simulink model "gm_ZynqBF_2tx_fpga"  (R2018b)
settings: Solver=FixedStepDiscrete  StartTime=0.0  StopTime=10.0  FixedStep=(1/420e3)/128  RelTol=1e-3
undefined symbols (not defined in the file or in its folder): a, b, c
libraries: hdlsllib x873, simulink x349
(part 3 of 40)

== system gm_ZynqBF_2tx_fpga/channel_estimator/gs_selector ==
  pd1 : Inport  OutDataTypeStr=boolean  PortDimensions=1  SampleTime=1.86011904761905e-08
  pd2 : Inport  Port=2  OutDataTypeStr=boolean  PortDimensions=1  SampleTime=1.86011904761905e-08
  en : Inport  Port=3  OutDataTypeStr=boolean  PortDimensions=1  SampleTime=1.86011904761905e-08
  Delay{1..5} (5 alike) : Delay  DelayLength=double(1)  InitialCondition=0  InputProcessing=Inherited  SampleTime=1.86011904761905e-08
  Switch1 : Switch  Criteria=u2 ~= 0  Threshold=double(0)  OutDataTypeStr=boolean  SampleTime=1.86011904761905e-08
  concatenate : Concatenate
  gs_sel : Outport
  wires:
  pd1/1 -> Delay1/1
  pd2/1 -> Delay2/1
  en/1 -> Delay4/1
  Delay1/1 -> concatenate/1
  Delay2/1 -> concatenate/2
  Delay3/1 -> gs_sel/1
  Delay4/1 -> Switch1/2
  Delay5/1 -> Switch1/3
  Switch1/1 -> Delay5/1, Delay3/1
  concatenate/1 -> Switch1/1

== system gm_ZynqBF_2tx_fpga/channel_estimator/in_fifo ==
  rxi_in : Inport  OutDataTypeStr=fixdt(1, 16, 15)  PortDimensions=1  SampleTime=2.38095238095238e-06
  rxq_in : Inport  Port=2  OutDataTypeStr=fixdt(1, 16, 15)  PortDimensions=1  SampleTime=2.38095238095238e-06
  rxv_in : Inport  Port=3  OutDataTypeStr=boolean  PortDimensions=1  SampleTime=2.38095238095238e-06
  pd_en : Inport  Port=4  OutDataTypeStr=boolean  PortDimensions=1  SampleTime=1.86011904761905e-08
  cf_en : Inport  Port=5  OutDataTypeStr=boolean  PortDimensions=1  SampleTime=1.86011904761905e-08
  Delay : Delay  DelayLength=double(1)  InitialCondition=0  InputProcessing=Inherited  SampleTime=2.38095238095238e-06
  Delay1 : Delay  DelayLength=double(1)  InitialCondition=0  InputProcessing=Inherited  SampleTime=2.38095238095238e-06
  Delay4 : Delay  DelayLength=double(2)  InitialCondition=0  InputProcessing=Inherited  SampleTime=1.86011904761905e-08
  Delay5 : Delay  DelayLength=double(1)  InitialCondition=0  InputProcessing=Inherited  SampleTime=1.86011904761905e-08
  Logical Operator : Logic  AllPortsSameDT=off  OutDataTypeStr=boolean  SampleTime=1.86011904761905e-08
  Logical Operator1 : Logic  AllPortsSameDT=off  OutDataTypeStr=boolean  SampleTime=2.38095238095238e-06
  Logical Operator2 : Logic  AllPortsSameDT=off  OutDataTypeStr=boolean  SampleTime=1.86011904761905e-08
  Logical Operator3 : Logic  Operator=NOR  AllPortsSameDT=off  OutDataTypeStr=boolean  SampleTime=1.86011904761905e-08
  Logical Operator4 : Logic  AllPortsSameDT=off  OutDataTypeStr=boolean  SampleTime=1.86011904761905e-08
  Logical Operator5 : Logic  Operator=OR  AllPortsSameDT=off  OutDataTypeStr=boolean  SampleTime=1.86011904761905e-08
  Rate Transition : RateTransition  InitialCondition=double(0)  OutPortSampleTimeOpt=Multiple of input port sample time  OutPortSampleTimeMultiple=128
  rx_i_fifo : hdlsllib/HDL RAMs/HDL FIFO  fifo_size=8912  ratio=1/128  push_msg=Warning  pop_msg=Warning  show_empty=on  show_full=off  show_num=off
      settings: SourceProductName=HDL Coder  SourceProductBaseCode=HD
  rx_q_fifo : hdlsllib/HDL RAMs/HDL FIFO  fifo_size=8912  ratio=1/128  push_msg=Warning  pop_msg=Warning  show_empty=on  show_full=off  show_num=off
      settings: SourceProductName=HDL Coder  SourceProductBaseCode=HD
  rxi_out : Outport
  rxq_out : Outport  Port=2
  rxv_out : Outport  Port=3
  empty : Outport  Port=4
  wires:
  rxi_in/1 -> Delay/1
  rxq_in/1 -> Delay1/1
  rxv_in/1 -> Logical Operator1/1
  pd_en/1 -> Logical Operator4/1, Rate Transition/1
  cf_en/1 -> Logical Operator2/1
  Delay/1 -> rx_i_fifo/1
  Delay1/1 -> rx_q_fifo/1
  Delay4/1 -> rxv_out/1
  Delay5/1 -> empty/1
  Logical Operator/1 -> Delay5/1
  Logical Operator1/1 -> rx_i_fifo/2, rx_q_fifo/2
  Logical Operator2/1 -> Logical Operator5/1
  Logical Operator3/1 -> Logical Operator4/2, Logical Operator2/2
  Logical Operator4/1 -> Logical Operator5/2, Delay4/1
  Logical Operator5/1 -> rx_i_fifo/3, rx_q_fifo/3
  Rate Transition/1 -> Logical Operator1/2
  rx_i_fifo/1 -> rxi_out/1
  rx_i_fifo/2 -> Logical Operator3/1, Logical Operator/1
  rx_q_fifo/1 -> rxq_out/1
  rx_q_fifo/2 -> Logical Operator3/2, Logical Operator/2

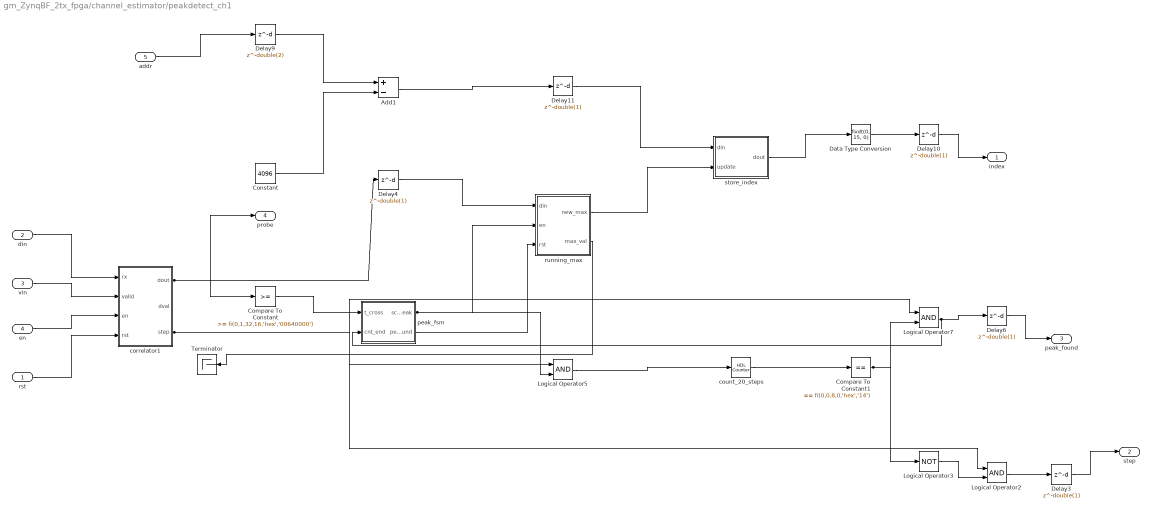
== system gm_ZynqBF_2tx_fpga/channel_estimator/peakdetect_ch1 ==
  rst : Inport  OutDataTypeStr=boolean  PortDimensions=1  SampleTime=1.86011904761905e-08
  din : Inport  Port=2  OutDataTypeStr=fixdt(1, 16, 15)  PortDimensions=[2]  SampleTime=1.86011904761905e-08
  vin : Inport  Port=3  OutDataTypeStr=boolean  PortDimensions=1  SampleTime=1.86011904761905e-08
  en : Inport  Port=4  OutDataTypeStr=boolean  PortDimensions=1  SampleTime=1.86011904761905e-08
  addr : Inport  Port=5  OutDataTypeStr=fixdt(0, 15, 0)  PortDimensions=1  SampleTime=1.86011904761905e-08
  Add1 : Sum  Inputs=+-  AccumDataTypeStr=fixdt(1, 17, 0)  OutDataTypeStr=int16  SampleTime=1.86011904761905e-08
  Compare To Constant : simulink/Logic and Bit Operations/Compare To Constant  relop=>=  const=fi(0,1,32,16,'hex','00640000')  OutDataTypeStr=boolean
  Compare To Constant1 : simulink/Logic and Bit Operations/Compare To Constant  relop===  const=fi(0,0,8,0,'hex','14')  OutDataTypeStr=boolean
  Constant : Constant  Value=4096  OutDataTypeStr=uint16  SampleTime=-1
  Data Type Conversion : DataTypeConversion  OutDataTypeStr=fixdt(0, 15, 0)  SampleTime=1.86011904761905e-08
  Delay{3..4,6,10..11} (5 alike) : Delay  DelayLength=double(1)  InitialCondition=0  InputProcessing=Inherited  SampleTime=1.86011904761905e-08
  Delay9 : Delay  DelayLength=double(2)  InitialCondition=0  InputProcessing=Inherited  SampleTime=1.86011904761905e-08
  Logical Operator2 : Logic  AllPortsSameDT=off  OutDataTypeStr=boolean  SampleTime=1.86011904761905e-08
  Logical Operator3 : Logic  Operator=NOT  Inputs=1  AllPortsSameDT=off  OutDataTypeStr=boolean  SampleTime=1.86011904761905e-08
  Logical Operator5 : Logic  AllPortsSameDT=off  OutDataTypeStr=boolean  SampleTime=1.86011904761905e-08
  Logical Operator7 : Logic  AllPortsSameDT=off  OutDataTypeStr=boolean  SampleTime=1.86011904761905e-08
  Terminator : Terminator
  correlator1 : Subsystem
  count_20_steps : hdlsllib/Sources/HDL Counter  CountType=Count limited  CountInit=double(0)  CountStep=double(1)  CountMax=double(20)  CountFromType=Initial value  CountFrom=double(0)  CountResetPort=off  CountLoadPort=off  CountEnbPort=on  CountDirPort=off  CountDataType=Unsigned  CountWordLen=8  CountFracLen=0  CountSampTime=1.86011904761905e-08
      settings: SourceProductBaseCode=HD
  peak_fsm : Subsystem
  running_max : Subsystem
  store_index : Subsystem
  index : Outport
  step : Outport  Port=2
  peak_found : Outport  Port=3
  probe : Outport  Port=4
  wires:
  rst/1 -> correlator1/4(rst)
  din/1 -> correlator1/1(rx)
  vin/1 -> correlator1/2(valid)
  en/1 -> correlator1/3(en)
  addr/1 -> Delay9/1
  Add1/1 -> Delay11/1
  Compare To Constant/1 -> peak_fsm/1(t_cross)
  Compare To Constant1/1 -> Logical Operator7/2, Logical Operator3/1
  Constant/1 -> Add1/2
  Data Type Conversion/1 -> Delay10/1
  Delay10/1 -> index/1
  Delay11/1 -> store_index/1(din)
  Delay3/1 -> step/1
  Delay4/1 -> running_max/1(din)
  Delay6/1 -> peak_found/1
  Delay9/1 -> Add1/1
  Logical Operator2/1 -> Delay3/1
  Logical Operator3/1 -> Logical Operator2/2
  Logical Operator5/1 -> count_20_steps/1
  Logical Operator7/1 -> Delay6/1, peak_fsm/2(cnt_end)
  correlator1/1(dout) -> Compare To Constant/1, Delay4/1, probe/1
  correlator1/3(step) -> Logical Operator7/1, Logical Operator5/1, Logical Operator2/1
  count_20_steps/1 -> Compare To Constant1/1
  peak_fsm/1(scan_peak) -> Logical Operator5/2, running_max/2(en)
  peak_fsm/2(peak_found) -> running_max/3(rst)
  running_max/1(new_max) -> store_index/2(update)
  running_max/2(max_val) -> Terminator/1
  store_index/1(dout) -> Data Type Conversion/1

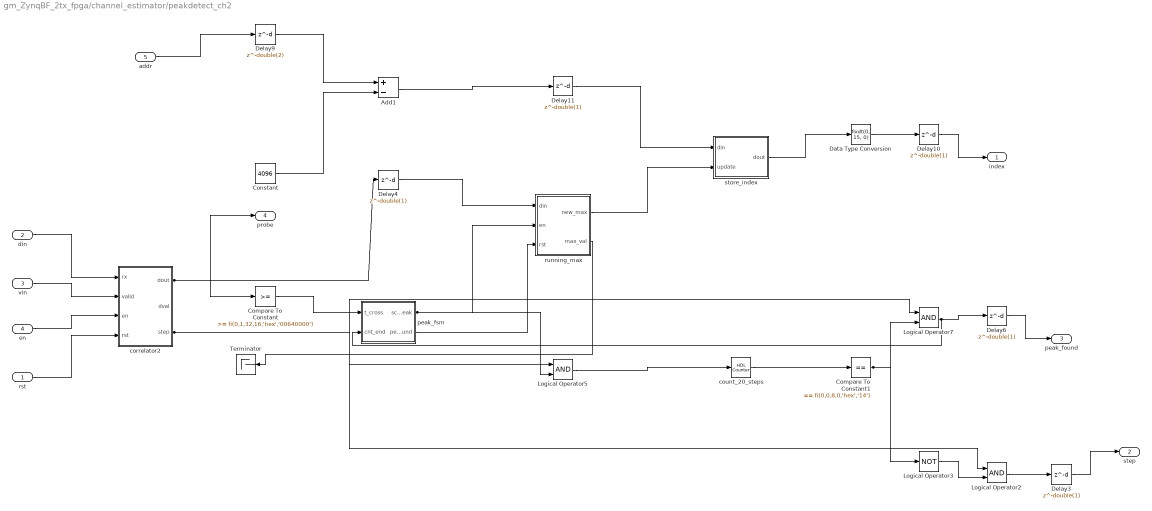
== system gm_ZynqBF_2tx_fpga/channel_estimator/peakdetect_ch2 ==
  rst : Inport  OutDataTypeStr=boolean  PortDimensions=1  SampleTime=1.86011904761905e-08
  din : Inport  Port=2  OutDataTypeStr=fixdt(1, 16, 15)  PortDimensions=[2]  SampleTime=1.86011904761905e-08
  vin : Inport  Port=3  OutDataTypeStr=boolean  PortDimensions=1  SampleTime=1.86011904761905e-08
  en : Inport  Port=4  OutDataTypeStr=boolean  PortDimensions=1  SampleTime=1.86011904761905e-08
  addr : Inport  Port=5  OutDataTypeStr=fixdt(0, 15, 0)  PortDimensions=1  SampleTime=1.86011904761905e-08
  Add1 : Sum  Inputs=+-  AccumDataTypeStr=fixdt(1, 17, 0)  OutDataTypeStr=int16  SampleTime=1.86011904761905e-08
  Compare To Constant : simulink/Logic and Bit Operations/Compare To Constant  relop=>=  const=fi(0,1,32,16,'hex','00640000')  OutDataTypeStr=boolean
  Compare To Constant1 : simulink/Logic and Bit Operations/Compare To Constant  relop===  const=fi(0,0,8,0,'hex','14')  OutDataTypeStr=boolean
  Constant : Constant  Value=4096  OutDataTypeStr=uint16  SampleTime=-1
  Data Type Conversion : DataTypeConversion  OutDataTypeStr=fixdt(0, 15, 0)  SampleTime=1.86011904761905e-08
  Delay{3..4,6,10..11} (5 alike) : Delay  DelayLength=double(1)  InitialCondition=0  InputProcessing=Inherited  SampleTime=1.86011904761905e-08
  Delay9 : Delay  DelayLength=double(2)  InitialCondition=0  InputProcessing=Inherited  SampleTime=1.86011904761905e-08
  Logical Operator2 : Logic  AllPortsSameDT=off  OutDataTypeStr=boolean  SampleTime=1.86011904761905e-08
  Logical Operator3 : Logic  Operator=NOT  Inputs=1  AllPortsSameDT=off  OutDataTypeStr=boolean  SampleTime=1.86011904761905e-08
  Logical Operator5 : Logic  AllPortsSameDT=off  OutDataTypeStr=boolean  SampleTime=1.86011904761905e-08
  Logical Operator7 : Logic  AllPortsSameDT=off  OutDataTypeStr=boolean  SampleTime=1.86011904761905e-08
  Terminator : Terminator
  correlator2 : Subsystem
  count_20_steps : hdlsllib/Sources/HDL Counter  CountType=Count limited  CountInit=double(0)  CountStep=double(1)  CountMax=double(20)  CountFromType=Initial value  CountFrom=double(0)  CountResetPort=off  CountLoadPort=off  CountEnbPort=on  CountDirPort=off  CountDataType=Unsigned  CountWordLen=8  CountFracLen=0  CountSampTime=1.86011904761905e-08
      settings: SourceProductBaseCode=HD
  peak_fsm : Subsystem
  running_max : Subsystem
  store_index : Subsystem
  index : Outport
  step : Outport  Port=2
  peak_found : Outport  Port=3
  probe : Outport  Port=4
  wires:
  rst/1 -> correlator2/4(rst)
  din/1 -> correlator2/1(rx)
  vin/1 -> correlator2/2(valid)
  en/1 -> correlator2/3(en)
  addr/1 -> Delay9/1
  Add1/1 -> Delay11/1
  Compare To Constant/1 -> peak_fsm/1(t_cross)
  Compare To Constant1/1 -> Logical Operator7/2, Logical Operator3/1
  Constant/1 -> Add1/2
  Data Type Conversion/1 -> Delay10/1
  Delay10/1 -> index/1
  Delay11/1 -> store_index/1(din)
  Delay3/1 -> step/1
  Delay4/1 -> running_max/1(din)
  Delay6/1 -> peak_found/1
  Delay9/1 -> Add1/1
  Logical Operator2/1 -> Delay3/1
  Logical Operator3/1 -> Logical Operator2/2
  Logical Operator5/1 -> count_20_steps/1
  Logical Operator7/1 -> Delay6/1, peak_fsm/2(cnt_end)
  correlator2/1(dout) -> Compare To Constant/1, Delay4/1, probe/1
  correlator2/3(step) -> Logical Operator7/1, Logical Operator5/1, Logical Operator2/1
  count_20_steps/1 -> Compare To Constant1/1
  peak_fsm/1(scan_peak) -> Logical Operator5/2, running_max/2(en)
  peak_fsm/2(peak_found) -> running_max/3(rst)
  running_max/1(new_max) -> store_index/2(update)
  running_max/2(max_val) -> Terminator/1
  store_index/1(dout) -> Data Type Conversion/1

== system gm_ZynqBF_2tx_fpga/channel_estimator/ram_counter ==
  rst : Inport  OutDataTypeStr=boolean  PortDimensions=1  SampleTime=1.86011904761905e-08
  ram_we : Inport  Port=2  OutDataTypeStr=boolean  PortDimensions=1  SampleTime=1.86011904761905e-08
  ram_re : Inport  Port=3  OutDataTypeStr=boolean  PortDimensions=1  SampleTime=1.86011904761905e-08
  pd_en : Inport  Port=4  OutDataTypeStr=boolean  PortDimensions=1  SampleTime=1.86011904761905e-08
  Compare To Constant : simulink/Logic and Bit Operations/Compare To Constant  relop=>  const=fi(0,0,16,0,'hex','0000')  OutDataTypeStr=boolean
  Compare To Constant1 : simulink/Logic and Bit Operations/Compare To Constant  relop===  const=fi(0,0,8,0,'hex','00')  OutDataTypeStr=boolean
  Delay{1,4..7} (5 alike) : Delay  DelayLength=double(1)  InitialCondition=0  InputProcessing=Inherited  SampleTime=1.86011904761905e-08
  Delay2 : Delay  DelayLength=double(4)  InitialCondition=0  InputProcessing=Inherited  SampleTime=1.86011904761905e-08
  Delay3 : Delay  DelayLength=double(4)  InitialCondition=0  InputProcessing=Inherited  SampleTime=1.86011904761905e-08
  HDL Counter : hdlsllib/Sources/HDL Counter  CountType=Free running  CountInit=double(0)  CountStep=double(1)  CountMax=25  CountFromType=Initial value  CountFrom=double(0)  CountResetPort=on  CountLoadPort=off  CountEnbPort=on  CountDirPort=on  CountDataType=Unsigned  CountWordLen=16  CountFracLen=0  CountSampTime=1.86011904761905e-08
      settings: SourceProductBaseCode=HD
  HDL Counter1 : hdlsllib/Sources/HDL Counter  CountType=Count limited  CountInit=double(0)  CountStep=double(1)  CountMax=double(1)  CountFromType=Initial value  CountFrom=double(0)  CountResetPort=on  CountLoadPort=off  CountEnbPort=on  CountDirPort=off  CountDataType=Unsigned  CountWordLen=8  CountFracLen=0  CountSampTime=1.86011904761905e-08
      settings: SourceProductBaseCode=HD
  Logical Operator : Logic  Operator=XOR  AllPortsSameDT=off  OutDataTypeStr=boolean  SampleTime=1.86011904761905e-08
  Logical Operator1 : Logic  AllPortsSameDT=off  OutDataTypeStr=boolean  SampleTime=1.86011904761905e-08
  Logical Operator2 : Logic  AllPortsSameDT=off  OutDataTypeStr=boolean  SampleTime=1.86011904761905e-08
  corr_en : Outport
  pd_init : Outport  Port=2
  wires:
  rst/1 -> Delay4/1
  ram_we/1 -> Delay1/1
  ram_re/1 -> Delay2/1
  pd_en/1 -> Delay3/1
  Compare To Constant/1 -> Delay6/1
  Compare To Constant1/1 -> Logical Operator2/2
  Delay1/1 -> Logical Operator2/1, Logical Operator/2, HDL Counter/3
  Delay2/1 -> Logical Operator1/2
  Delay3/1 -> Logical Operator1/1
  Delay4/1 -> HDL Counter1/1, HDL Counter/1
  Delay5/1 -> Logical Operator/1
  Delay6/1 -> corr_en/1
  Delay7/1 -> pd_init/1
  HDL Counter/1 -> Compare To Constant/1
  HDL Counter1/1 -> Compare To Constant1/1
  Logical Operator/1 -> HDL Counter/2
  Logical Operator1/1 -> Delay5/1
  Logical Operator2/1 -> HDL Counter1/2, Delay7/1

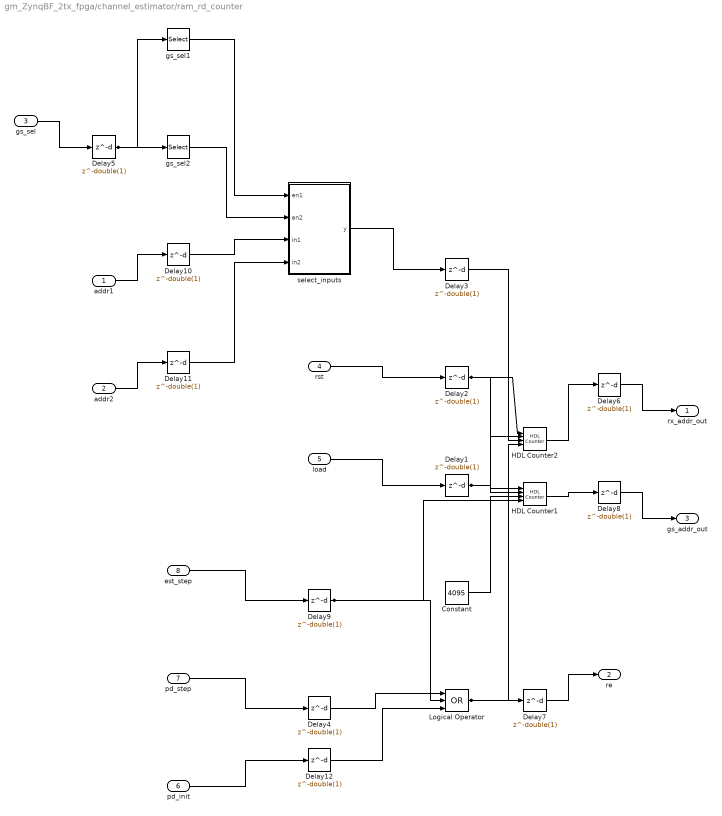
== system gm_ZynqBF_2tx_fpga/channel_estimator/ram_rd_counter ==
  addr1 : Inport  OutDataTypeStr=fixdt(0, 15, 0)  PortDimensions=1  SampleTime=1.86011904761905e-08
  addr2 : Inport  Port=2  OutDataTypeStr=fixdt(0, 15, 0)  PortDimensions=1  SampleTime=1.86011904761905e-08
  gs_sel : Inport  Port=3  OutDataTypeStr=boolean  PortDimensions=[2]  SampleTime=1.86011904761905e-08
  rst : Inport  Port=4  OutDataTypeStr=boolean  PortDimensions=1  SampleTime=1.86011904761905e-08
  load : Inport  Port=5  OutDataTypeStr=boolean  PortDimensions=1  SampleTime=1.86011904761905e-08
  pd_init : Inport  Port=6  OutDataTypeStr=boolean  PortDimensions=1  SampleTime=1.86011904761905e-08
  pd_step : Inport  Port=7  OutDataTypeStr=boolean  PortDimensions=1  SampleTime=1.86011904761905e-08
  est_step : Inport  Port=8  OutDataTypeStr=boolean  PortDimensions=1  SampleTime=1.86011904761905e-08
  Constant : Constant  Value=4095  OutDataTypeStr=fixdt(0, 12, 0)  SampleTime=-1
  Delay{1..12} (12 alike) : Delay  DelayLength=double(1)  InitialCondition=0  InputProcessing=Inherited  SampleTime=1.86011904761905e-08
  HDL Counter1 : hdlsllib/Sources/HDL Counter  CountType=Count limited  CountInit=double(0)  CountStep=double(1)  CountMax=double(4095)  CountFromType=Initial value  CountFrom=double(0)  CountResetPort=on  CountLoadPort=on  CountEnbPort=on  CountDirPort=off  CountDataType=Unsigned  CountWordLen=12  CountFracLen=0  CountSampTime=1.86011904761905e-08
      settings: SourceProductBaseCode=HD
  HDL Counter2 : hdlsllib/Sources/HDL Counter  CountType=Count limited  CountInit=double(0)  CountStep=double(1)  CountMax=double(32767)  CountFromType=Initial value  CountFrom=double(0)  CountResetPort=on  CountLoadPort=on  CountEnbPort=on  CountDirPort=off  CountDataType=Unsigned  CountWordLen=15  CountFracLen=0  CountSampTime=1.86011904761905e-08
      settings: SourceProductBaseCode=HD
  Logical Operator : Logic  Operator=OR  Inputs=3  AllPortsSameDT=off  OutDataTypeStr=boolean  SampleTime=1.86011904761905e-08
  gs_sel1 : Selector  IndexMode=Zero-based  SampleTime=1.86011904761905e-08  IndexOptions=Index vector (dialog)  Indices=double(0)  OutputSizes=double(1)
  gs_sel2 : Selector  IndexMode=Zero-based  SampleTime=1.86011904761905e-08  IndexOptions=Index vector (dialog)  Indices=double(1)  OutputSizes=double(1)
  select_inputs : Subsystem
  rx_addr_out : Outport
  re : Outport  Port=2
  gs_addr_out : Outport  Port=3
  wires:
  addr1/1 -> Delay10/1
  addr2/1 -> Delay11/1
  gs_sel/1 -> Delay5/1
  rst/1 -> Delay2/1
  load/1 -> Delay1/1
  pd_init/1 -> Delay12/1
  pd_step/1 -> Delay4/1
  est_step/1 -> Delay9/1
  Constant/1 -> HDL Counter1/3
  Delay1/1 -> HDL Counter2/2, HDL Counter1/2
  Delay10/1 -> select_inputs/3(in1)
  Delay11/1 -> select_inputs/4(in2)
  Delay12/1 -> Logical Operator/3
  Delay2/1 -> HDL Counter2/1, HDL Counter1/1
  Delay3/1 -> HDL Counter2/3
  Delay4/1 -> Logical Operator/1
  Delay5/1 -> gs_sel2/1, gs_sel1/1
  Delay6/1 -> rx_addr_out/1
  Delay7/1 -> re/1
  Delay8/1 -> gs_addr_out/1
  Delay9/1 -> Logical Operator/2, HDL Counter1/4
  HDL Counter1/1 -> Delay8/1
  HDL Counter2/1 -> Delay6/1
  Logical Operator/1 -> HDL Counter2/4, Delay7/1
  gs_sel1/1 -> select_inputs/1(en1)
  gs_sel2/1 -> select_inputs/2(en2)
  select_inputs/1(y) -> Delay3/1

== system gm_ZynqBF_2tx_fpga/channel_estimator/rx_bram ==
  din_i : Inport  OutDataTypeStr=fixdt(1, 16, 15)  PortDimensions=1  SampleTime=1.86011904761905e-08
  din_q : Inport  Port=2  OutDataTypeStr=fixdt(1, 16, 15)  PortDimensions=1  SampleTime=1.86011904761905e-08
  we : Inport  Port=3  OutDataTypeStr=boolean  PortDimensions=1  SampleTime=1.86011904761905e-08
  re : Inport  Port=4  OutDataTypeStr=boolean  PortDimensions=1  SampleTime=1.86011904761905e-08
  rd_addr : Inport  Port=5  OutDataTypeStr=fixdt(0, 15, 0)  PortDimensions=1  SampleTime=1.86011904761905e-08
  rst : Inport  Port=6  OutDataTypeStr=boolean  PortDimensions=1  SampleTime=1.86011904761905e-08
  Delay{1..4,6..7} (6 alike) : Delay  DelayLength=double(1)  InitialCondition=0  InputProcessing=Inherited  SampleTime=1.86011904761905e-08
  Delay5 : Delay  DelayLength=double(4)  InitialCondition=0  InputProcessing=Inherited  SampleTime=1.86011904761905e-08
  Delay8 : Delay  DelayLength=double(4)  InitialCondition=0  InputProcessing=Inherited  SampleTime=1.86011904761905e-08
  HDL Counter : hdlsllib/Sources/HDL Counter  CountType=Count limited  CountInit=double(1)  CountStep=double(1)  CountMax=double(32767)  CountFromType=Initial value  CountFrom=double(1)  CountResetPort=on  CountLoadPort=off  CountEnbPort=on  CountDirPort=off  CountDataType=Unsigned  CountWordLen=15  CountFracLen=0  CountSampTime=1.86011904761905e-08
      settings: SourceProductBaseCode=HD
  concatenate : Concatenate
  rx_ram_i : hdlsllib/HDL RAMs/Simple Dual Port RAM  ram_size=15
      settings: SourceProductName=HDL Coder  SourceProductBaseCode=HD
  rx_ram_q : hdlsllib/HDL RAMs/Simple Dual Port RAM  ram_size=15
      settings: SourceProductName=HDL Coder  SourceProductBaseCode=HD
  dout : Outport
  valid : Outport  Port=2
  addr_out : Outport  Port=3
  wires:
  din_i/1 -> Delay3/1
  din_q/1 -> Delay4/1
  we/1 -> Delay1/1
  re/1 -> Delay5/1
  rd_addr/1 -> Delay8/1, Delay2/1
  rst/1 -> HDL Counter/1
  Delay1/1 -> HDL Counter/2, rx_ram_i/3, rx_ram_q/3
  Delay2/1 -> rx_ram_i/4, rx_ram_q/4
  Delay3/1 -> rx_ram_i/1
  Delay4/1 -> rx_ram_q/1
  Delay5/1 -> valid/1
  Delay6/1 -> concatenate/1
  Delay7/1 -> concatenate/2
  Delay8/1 -> addr_out/1
  HDL Counter/1 -> rx_ram_i/2, rx_ram_q/2
  concatenate/1 -> dout/1
  rx_ram_i/1 -> Delay6/1
  rx_ram_q/1 -> Delay7/1

== system gm_ZynqBF_2tx_fpga/channel_estimator/state_machine ==
  peak_found : Inport  OutDataTypeStr=boolean  PortDimensions=1  SampleTime=1.86011904761905e-08
  est_done : Inport  Port=2  OutDataTypeStr=boolean  PortDimensions=1  SampleTime=1.86011904761905e-08
  cf_done : Inport  Port=3  OutDataTypeStr=boolean  PortDimensions=1  SampleTime=1.86011904761905e-08
  Compare To Constant : simulink/Logic and Bit Operations/Compare To Constant  relop===  const=fi(0,0,8,0,'hex','00')  OutDataTypeStr=boolean
  Compare To Constant1 : simulink/Logic and Bit Operations/Compare To Constant  relop===  const=fi(0,0,8,0,'hex','01')  OutDataTypeStr=boolean
  Compare To Constant2 : simulink/Logic and Bit Operations/Compare To Constant  relop===  const=fi(0,0,8,0,'hex','02')  OutDataTypeStr=boolean
  Delay : Delay  DelayLength=double(3)  InitialCondition=0  InputProcessing=Inherited  SampleTime=1.86011904761905e-08
  Delay1 : Delay  DelayLength=double(3)  InitialCondition=0  InputProcessing=Inherited  SampleTime=1.86011904761905e-08
  HDL Counter : hdlsllib/Sources/HDL Counter  CountType=Count limited  CountInit=double(0)  CountStep=double(1)  CountMax=double(2)  CountFromType=Initial value  CountFrom=double(0)  CountResetPort=off  CountLoadPort=off  CountEnbPort=on  CountDirPort=off  CountDataType=Unsigned  CountWordLen=8  CountFracLen=0  CountSampTime=1.86011904761905e-08
      settings: SourceProductBaseCode=HD
  Logical Operator1 : Logic  AllPortsSameDT=off  OutDataTypeStr=boolean  SampleTime=1.86011904761905e-08
  Logical Operator3 : Logic  Operator=OR  Inputs=3  AllPortsSameDT=off  OutDataTypeStr=boolean  SampleTime=1.86011904761905e-08
  pd_en : Outport
  est_en : Outport  Port=2
  cf_en : Outport  Port=3
  probe_state : Outport  Port=4
  wires:
  peak_found/1 -> Delay/1
  est_done/1 -> Delay1/1
  cf_done/1 -> Logical Operator1/1
  Compare To Constant/1 -> pd_en/1
  Compare To Constant1/1 -> est_en/1
  Compare To Constant2/1 -> Logical Operator1/2, cf_en/1
  Delay/1 -> Logical Operator3/1
  Delay1/1 -> Logical Operator3/2
  HDL Counter/1 -> Compare To Constant2/1, Compare To Constant1/1, Compare To Constant/1, probe_state/1
  Logical Operator1/1 -> Logical Operator3/3
  Logical Operator3/1 -> HDL Counter/1

== system gm_ZynqBF_2tx_fpga/channel_estimator/ch_est/calc_inverse ==
  din : Inport  OutDataTypeStr=fixdt(1, 32, 16)  PortDimensions=1  SampleTime=1.86011904761905e-08
  en : Inport  Port=2  OutDataTypeStr=boolean  PortDimensions=1  SampleTime=1.86011904761905e-08
  Compare To Constant : simulink/Logic and Bit Operations/Compare To Constant  relop===  const=fi(0,0,8,0,'hex','04')  OutDataTypeStr=boolean
  Delay18 : Delay  DelayLength=double(1)  InitialCondition=0  InputProcessing=Inherited  SampleTime=1.86011904761905e-08
  Delay20 : Delay  DelayLength=double(1)  InitialCondition=0  InputProcessing=Inherited  SampleTime=1.86011904761905e-08
  Delay4 : Delay  DelayLength=double(1)  InitialCondition=0  InputProcessing=Inherited  SampleTime=1.86011904761905e-08
  HDL Counter : hdlsllib/Sources/HDL Counter  CountType=Count limited  CountInit=double(0)  CountStep=double(1)  CountMax=double(9)  CountFromType=Initial value  CountFrom=double(0)  CountResetPort=on  CountLoadPort=off  CountEnbPort=on  CountDirPort=off  CountDataType=Unsigned  CountWordLen=8  CountFracLen=0  CountSampTime=1.86011904761905e-08
      settings: SourceProductBaseCode=HD
  HDL Reciprocal : Subsystem
  Logical Operator2 : Logic  Operator=NOT  Inputs=1  AllPortsSameDT=off  OutDataTypeStr=boolean  SampleTime=1.86011904761905e-08
  Switch1 : Switch  Criteria=u2 ~= 0  Threshold=double(0)  OutDataTypeStr=fixdt(1, 32, 14)  SampleTime=1.86011904761905e-08
  dout : Outport
  dval : Outport  Port=2
  wires:
  din/1 -> HDL Reciprocal/1(In1)
  en/1 -> Logical Operator2/1, HDL Counter/2
  Compare To Constant/1 -> Switch1/2, Delay18/1
  Delay18/1 -> dval/1
  Delay20/1 -> dout/1
  Delay4/1 -> Switch1/3
  HDL Counter/1 -> Compare To Constant/1
  HDL Reciprocal/1(Out1) -> Switch1/1
  Logical Operator2/1 -> HDL Counter/1
  Switch1/1 -> Delay4/1, Delay20/1

== system gm_ZynqBF_2tx_fpga/channel_estimator/ch_est/local_fsm ==
  nr_done : Inport  OutDataTypeStr=boolean  PortDimensions=1  SampleTime=1.86011904761905e-08
  dp_done : Inport  Port=2  OutDataTypeStr=boolean  PortDimensions=1  SampleTime=1.86011904761905e-08
  Compare To Constant : simulink/Logic and Bit Operations/Compare To Constant  relop===  const=fi(0,0,8,0,'hex','00')  OutDataTypeStr=boolean
  Compare To Constant1 : simulink/Logic and Bit Operations/Compare To Constant  relop===  const=fi(0,0,8,0,'hex','01')  OutDataTypeStr=boolean
  Compare To Constant2 : simulink/Logic and Bit Operations/Compare To Constant  relop===  const=fi(0,0,8,0,'hex','02')  OutDataTypeStr=boolean
  HDL Counter : hdlsllib/Sources/HDL Counter  CountType=Count limited  CountInit=double(0)  CountStep=double(1)  CountMax=double(2)  CountFromType=Initial value  CountFrom=double(0)  CountResetPort=off  CountLoadPort=off  CountEnbPort=on  CountDirPort=off  CountDataType=Unsigned  CountWordLen=8  CountFracLen=0  CountSampTime=1.86011904761905e-08
      settings: SourceProductBaseCode=HD
  Logical Operator : Logic  Operator=OR  Inputs=3  AllPortsSameDT=off  OutDataTypeStr=boolean  SampleTime=1.86011904761905e-08
  en_dp : Outport
  en_nr : Outport  Port=2
  en_est : Outport  Port=3
  wires:
  nr_done/1 -> Logical Operator/2
  dp_done/1 -> Logical Operator/1
  Compare To Constant/1 -> en_dp/1
  Compare To Constant1/1 -> en_nr/1
  Compare To Constant2/1 -> Logical Operator/3, en_est/1
  HDL Counter/1 -> Compare To Constant2/1, Compare To Constant1/1, Compare To Constant/1
  Logical Operator/1 -> HDL Counter/1

== system gm_ZynqBF_2tx_fpga/channel_estimator/ch_est/select_inputs ==
  en1 : Inport  OutDataTypeStr=boolean  PortDimensions=1  SampleTime=1.86011904761905e-08
  en2 : Inport  Port=2  OutDataTypeStr=boolean  PortDimensions=1  SampleTime=1.86011904761905e-08
  in1 : Inport  Port=3  OutDataTypeStr=fixdt(1, 16, 15)  PortDimensions=[2]  SampleTime=1.86011904761905e-08
  in2 : Inport  Port=4  OutDataTypeStr=fixdt(1, 16, 15)  PortDimensions=[2]  SampleTime=1.86011904761905e-08
  select_inputs : MATLAB Function  TreatAsAtomicUnit=on
  y : Outport
  wires:
  en1/1 -> select_inputs/1(en1)
  en2/1 -> select_inputs/2(en2)
  in1/1 -> select_inputs/3(in1)
  in2/1 -> select_inputs/4(in2)
  select_inputs/1(y) -> y/1

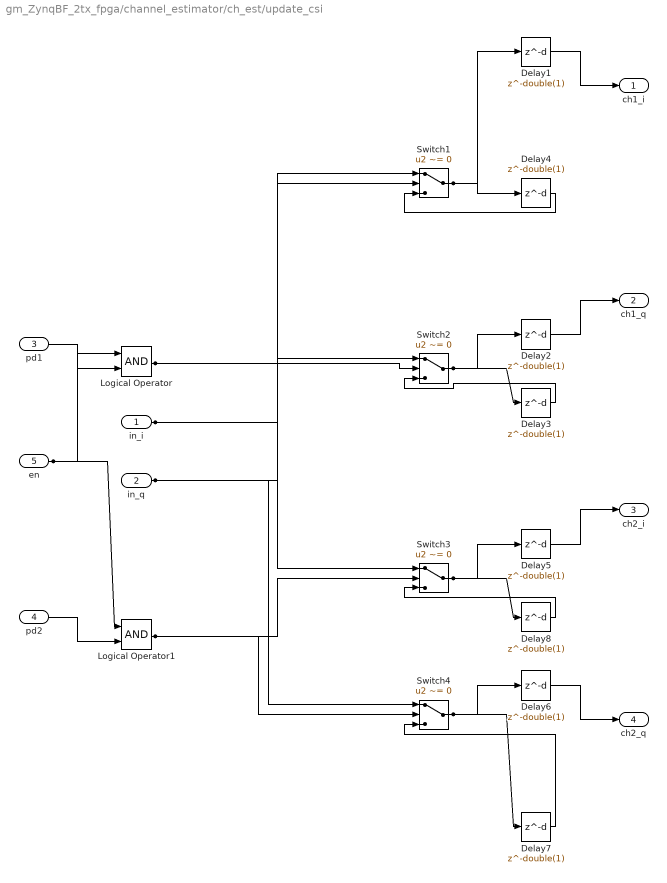
== system gm_ZynqBF_2tx_fpga/channel_estimator/ch_est/update_csi ==
  in_i : Inport  OutDataTypeStr=fixdt(1, 16, 15)  PortDimensions=1  SampleTime=1.86011904761905e-08
  in_q : Inport  Port=2  OutDataTypeStr=fixdt(1, 16, 15)  PortDimensions=1  SampleTime=1.86011904761905e-08
  pd1 : Inport  Port=3  OutDataTypeStr=boolean  PortDimensions=1  SampleTime=1.86011904761905e-08
  pd2 : Inport  Port=4  OutDataTypeStr=boolean  PortDimensions=1  SampleTime=1.86011904761905e-08
  en : Inport  Port=5  OutDataTypeStr=boolean  PortDimensions=1  SampleTime=1.86011904761905e-08
  Delay{1..8} (8 alike) : Delay  DelayLength=double(1)  InitialCondition=0  InputProcessing=Inherited  SampleTime=1.86011904761905e-08
  Logical Operator : Logic  AllPortsSameDT=off  OutDataTypeStr=boolean  SampleTime=1.86011904761905e-08
  Logical Operator1 : Logic  AllPortsSameDT=off  OutDataTypeStr=boolean  SampleTime=1.86011904761905e-08
  Switch{1..4} (4 alike) : Switch  Criteria=u2 ~= 0  Threshold=double(0)  OutDataTypeStr=fixdt(1, 16, 15)  SampleTime=1.86011904761905e-08
  ch1_i : Outport
  ch1_q : Outport  Port=2
  ch2_i : Outport  Port=3
  ch2_q : Outport  Port=4
  wires:
  in_i/1 -> Switch3/1, Switch1/1
  in_q/1 -> Switch4/1, Switch2/1
  pd1/1 -> Logical Operator/2
  pd2/1 -> Logical Operator1/2
  en/1 -> Logical Operator1/1, Logical Operator/1
  Delay1/1 -> ch1_i/1
  Delay2/1 -> ch1_q/1
  Delay3/1 -> Switch2/3
  Delay4/1 -> Switch1/3
  Delay5/1 -> ch2_i/1
  Delay6/1 -> ch2_q/1
  Delay7/1 -> Switch4/3
  Delay8/1 -> Switch3/3
  Logical Operator/1 -> Switch2/2, Switch1/2
  Logical Operator1/1 -> Switch4/2, Switch3/2
  Switch1/1 -> Delay4/1, Delay1/1
  Switch2/1 -> Delay3/1, Delay2/1
  Switch3/1 -> Delay8/1, Delay5/1
  Switch4/1 -> Delay7/1, Delay6/1
